simulink model "ExpCtrl"  (R2013a)
settings: Solver=ode45  StartTime=0.0  StopTime=10.0  RelTol=1e-3
values from neighbouring files (symbols this model uses):
  x0 = [0;0;0;0]    [SimModelMLD.m]
undefined symbols (not defined in the file or in its folder): model
libraries: mpt_sim x1
settings Model: Creator=root  LastModifiedBy=root

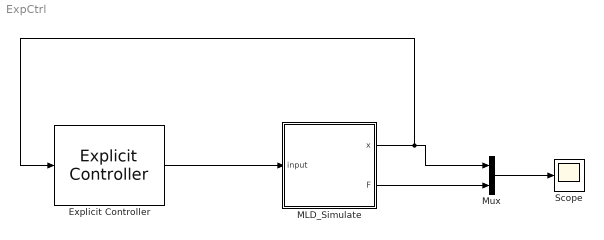
== system ExpCtrl ==
  Explicit Controller : mpt_sim/Explicit Controller
  MLD_Simulate : Subsystem
  Mux : Mux  Inputs=2
  Scope : Scope
  wires:
  Explicit Controller/1 -> MLD_Simulate/1(input)
  MLD_Simulate/1(x) -> Explicit Controller/1, Mux/1
  MLD_Simulate/2(F) -> Mux/2
  Mux/1 -> Scope/1

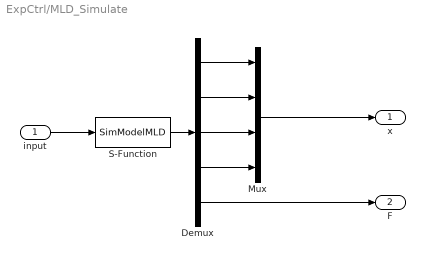
== system ExpCtrl/MLD_Simulate ==
  input : Inport
  Demux : Demux  Outputs=5
  Mux : Mux
  S-Function : S-Function  FunctionName=SimModelMLD  Parameters=model,x0  EnableBusSupport=off
  x : Outport
  F : Outport  Port=2
  wires:
  input/1 -> S-Function/1
  S-Function/1 -> Demux/1
  Demux/5 -> F/1
  Demux/3 -> Mux/3
  Demux/4 -> Mux/4
  Demux/1 -> Mux/1
  Demux/2 -> Mux/2
  Mux/1 -> x/1
